simulink model "ADCS_Design_RJF_Linear"  (R2024b)
settings: Solver=VariableStepAuto  StartTime=0.0  StopTime=tspan  FixedStep=10  RelTol=1e-4
values from neighbouring files (symbols this model uses):
  E_b_ECI_0 = C2EulerAngles(C_b_ECI_0)    [Final_Project_Part_2_init_Template.m]
  q_b_ECI_0 = C2quat(C_b_ECI_0)    [Final_Project_Part_2_init_Template.m]
  T = [0;0;0]    [Final_Project_Part_2_init_Template.m]
  w_b_ECI_0 = [0.001; -0.001; 0.002]    [Final_Project_Part_2_init_Template.m]
undefined symbols (not defined in the file or in its folder): J, Kd, Kp, q_C
settings Model: Creator=emehiel  LastModifiedBy=rosha
settings SolverCC: AlgebraicLoopSolver=TrustRegion
settings DebuggingCC: UnconnectedInputMsg=warning  UnconnectedOutputMsg=warning  UnconnectedLineMsg=warning
settings ModelReferenceCC: EnableRefExpFcnMdlSchedulingChecks=on
settings RTWCC: GPUComputeCapability=3.5

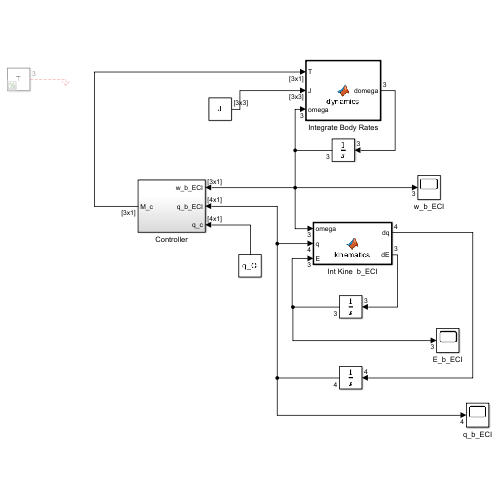
[thumbnail: Simulink's stored preview of the top-level diagram]
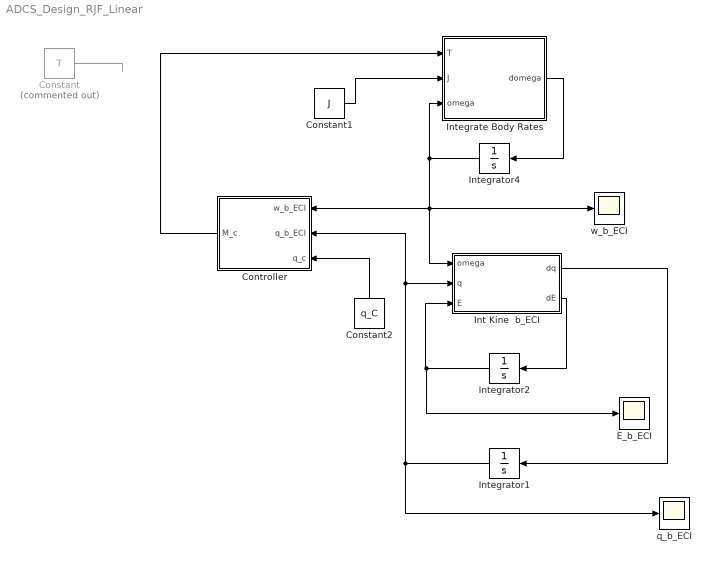
== system ADCS_Design_RJF_Linear ==
  Constant : Constant  Commented=on  Value=T
  Constant1 : Constant  Value=J
  Constant2 : Constant  Value=q_C
  Controller : Subsystem
  E_b_ECI : Scope
  Int Kine  b_ECI : MATLAB Function  TreatAsAtomicUnit=on
  Integrate Body Rates : MATLAB Function  TreatAsAtomicUnit=on
  Integrator1 : Integrator  InitialCondition=q_b_ECI_0
  Integrator2 : Integrator  InitialCondition=E_b_ECI_0
  Integrator4 : Integrator  InitialCondition=w_b_ECI_0
  q_b_ECI : Scope
  w_b_ECI : Scope
  wires:
  Constant/1 -> ?
  Constant1/1 -> Integrate Body Rates/2(J)
  Integrate Body Rates/1(domega) -> Integrator4/1
  Integrator4/1 -> w_b_ECI/1, Controller/1(w_b_ECI), Int Kine  b_ECI/1(omega), Integrate Body Rates/3(omega)
  Integrator2/1 -> E_b_ECI/1, Int Kine  b_ECI/3(E)
  Int Kine  b_ECI/2(dE) -> Integrator2/1
  Int Kine  b_ECI/1(dq) -> Integrator1/1
  Controller/1(M_c) -> Integrate Body Rates/1(T)
  Integrator1/1 -> q_b_ECI/1, Controller/2(q_b_ECI), Int Kine  b_ECI/2(q)
  Constant2/1 -> Controller/3(q_c)

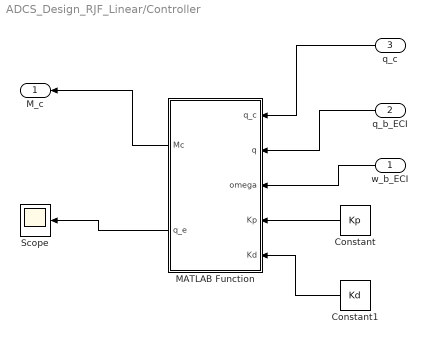
== system ADCS_Design_RJF_Linear/Controller ==
  w_b_ECI : Inport  PortDimensions=[3 1]
  q_b_ECI : Inport  Port=2  PortDimensions=[4 1]
  q_c : Inport  Port=3  PortDimensions=[4 1]
  Constant : Constant  Value=Kp
  Constant1 : Constant  Value=Kd
  MATLAB Function : MATLAB Function  TreatAsAtomicUnit=on
  Scope : Scope
  M_c : Outport  PortDimensions=[3 1]  VectorParamsAs1DForOutWhenUnconnected=off
  wires:
  MATLAB Function/1(Mc) -> M_c/1
  q_c/1 -> MATLAB Function/1(q_c)
  q_b_ECI/1 -> MATLAB Function/2(q)
  w_b_ECI/1 -> MATLAB Function/3(omega)
  Constant/1 -> MATLAB Function/4(Kp)
  Constant1/1 -> MATLAB Function/5(Kd)
  MATLAB Function/2(q_e) -> Scope/1

== matlab function ADCS_Design_RJF_Linear/Int Kine  b_ECI ==
  data: omega input; q input; dq output; E input; dE output
function [dq,dE] = kinematics(omega, q, E)
%#codegen

% unpack quaternion

epsilon = q(1:3,1);
eta = q(4,1);

depsilon = 1/2*(eta*eye(3) + vcross(epsilon))*omega;
deta = -1/2*epsilon'*omega;

dq = [depsilon; deta];

LBI = 1/cos(E(2))*[cos(E(2)) sin(E(1))*sin(E(2))  cos(E(1))*sin(E(2));
                   0         cos(E(1))*cos(E(2)) -sin(E(1))*cos(E(2));
                   0         sin(E(1))            cos(E(1))];

dE = LBI*omega;

== matlab function ADCS_Design_RJF_Linear/Integrate Body Rates ==
  data: T input; J input; omega input; domega output
function domega = dynamics(T, J, omega)
%#codegen

domega = J\(T - cross(omega, J*omega));

== matlab function ADCS_Design_RJF_Linear/Controller/MATLAB Function ==
  data: q_c input; Mc output; q input; omega input; Kp input; Kd input; q_e output
function [Mc,q_e]  = control_law(q_c, q, omega, Kp, Kd)
%#codegen

%q_e = quatMult(quatConjugate(q_c), q);
q_e = quatMult(q, quatConjugate(q_c));
Mc = -Kp*q_e(1:3,1) - Kd*omega;
